simulink model "Simscape_assignment"  (R2022a)
settings: Solver=VariableStepAuto  StartTime=0.0  StopTime=10.0  RelTol=1e-3
values from neighbouring files (symbols this model uses):
  c1 = 1500    [main.m]
  c2 = c1    (= 1500)    [main.m]
  V = 20/3.6    (= 5.55555555556)    [main.m]
libraries: fl_lib x20, nesl_utility x11, sdl_lib x4, cstblocks x1, motdrv_lib x1
settings Model: Creator=s393429  LastModifiedBy=s393429

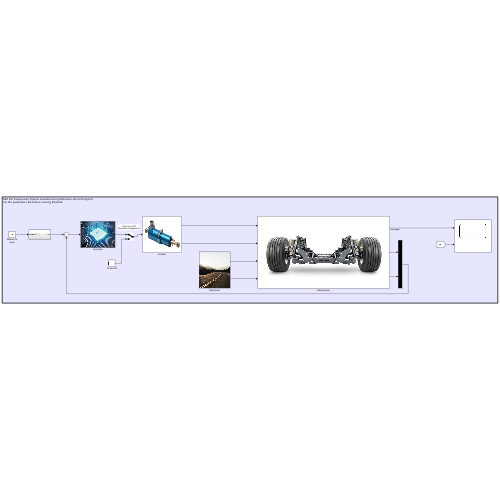
[thumbnail: Simulink's stored preview of the top-level diagram]
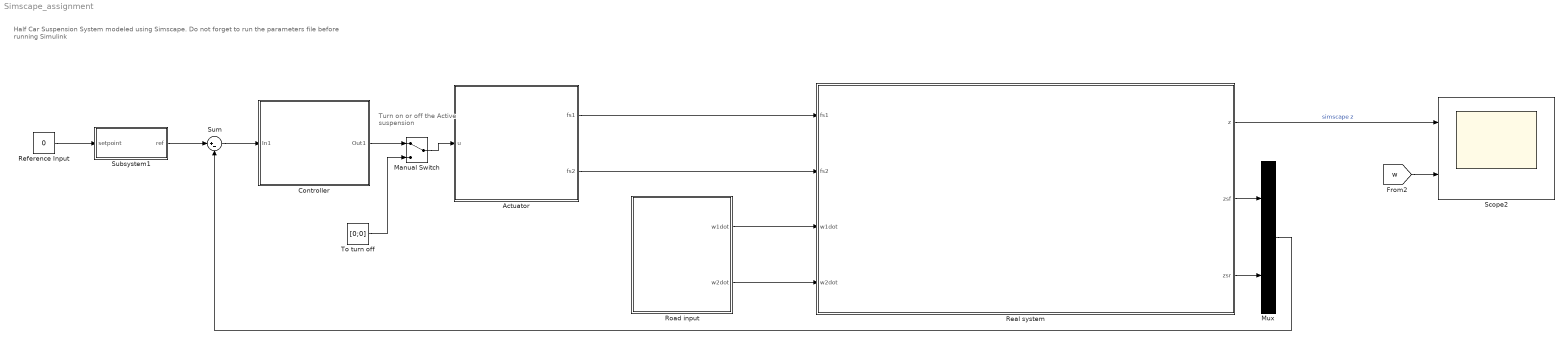
== system Simscape_assignment ==
  note: Half Car Suspension System modeled using Simscape. Do not forget to
      | run the parameters file before running Simulink
  note: Turn on or off
      | the Active suspension
  Actuator : Subsystem
      mask Display: image('actuator.jpg'); % Use "Edit Image" on toolstrip to change.
  Controller : Subsystem
      mask Display: image('cu.jpg'); % Use "Edit Image" on toolstrip to change.
  Manual Switch : ManualSwitch
  Mux : Mux  Inputs=2
  Real system : Subsystem
      mask Display: image('susp.jpg'); % Use "Edit Image" on toolstrip to change.
  Reference Input : Constant  Value=0
  Road input : Subsystem
      mask Display: image('road.jpg'); % Use "Edit Image" on toolstrip to change.
  Scope2 : Scope  NumInputPorts=2
  Subsystem1 : Subsystem
  Sum : Sum  Inputs=|+-
  To turn off : Constant  Value=[0;0]
  wires:
  Actuator/2(fs2) -> Real system/2(fs2)
  Actuator/1(fs1) -> Real system/1(fs1)
  [w] -> Scope2/2
  Real system/2(zsf) -> Mux/1
  Reference Input/1 -> Subsystem1/1(setpoint)
  Real system/3(zsr) -> Mux/2
  Road input/1(w1dot) -> Real system/3(w1dot)
  Sum/1 -> Controller/1(In1)
  Mux/1 -> Sum/2
  Subsystem1/1(ref) -> Sum/1
  Road input/2(w2dot) -> Real system/4(w2dot)
  Real system/1(z) -> Scope2/1  "simscape z"
  Controller/1(Out1) -> Manual Switch/1
  Manual Switch/1 -> Actuator/1(u)
  To turn off/1 -> Manual Switch/2

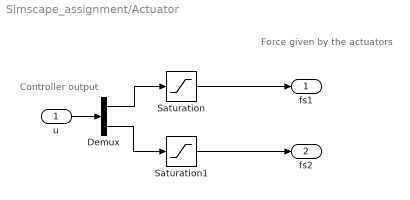
== system Simscape_assignment/Actuator ==
  note: Force given by
      | the actuators
  note: Controller output
  u : Inport
  Demux : Demux  Outputs=2
  Saturation : Saturate  UpperLimit=1e4  LowerLimit=-1e4
  Saturation1 : Saturate  UpperLimit=1e4  LowerLimit=-1e4
  fs1 : Outport
  fs2 : Outport  Port=2
  wires:
  u/1 -> Demux/1
  Demux/1 -> Saturation/1
  Saturation/1 -> fs1/1
  Demux/2 -> Saturation1/1
  Saturation1/1 -> fs2/1

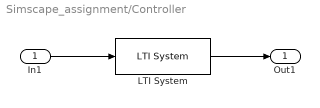
== system Simscape_assignment/Controller ==
  In1 : Inport
  LTI System : cstblocks/LTI System  sys=C  IC=[]
  Out1 : Outport
  wires:
  In1/1 -> LTI System/1
  LTI System/1 -> Out1/1

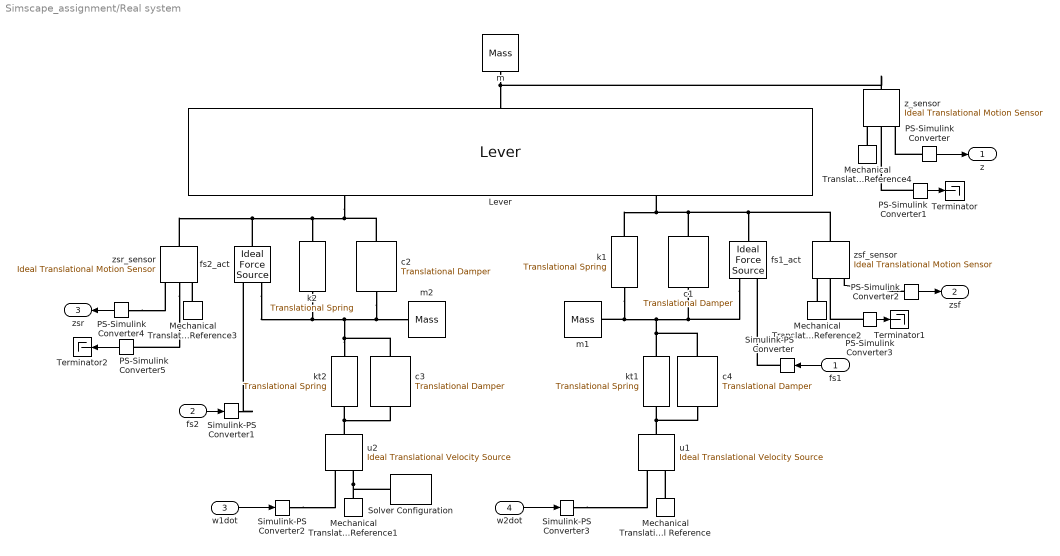
== system Simscape_assignment/Real system ==
  fs1 : Inport
  fs2 : Inport  Port=2
  w1dot : Inport  Port=3
  w2dot : Inport  Port=4
  Lever : fl_lib/Mechanical/Mechanisms/Lever  arm_AC=ar m  arm_BC=af m  f_A_specify=off  f_A_priority=None  f_A=0 N  f_A_nominal_specify=off  f_A_nominal_unit=N  f_A_nominal_value=1  f_B_specify=off  f_B_priority=None  f_B=0 N  f_B_nominal_specify=off  f_B_nominal_unit=N  f_B_nominal_value=1  f_C_specify=off  f_C_priority=None  f_C=0 N  f_C_nominal_specify=off  f_C_nominal_unit=N  f_C_nominal_value=1
      settings: SourceProductBaseCode=PW,SS,VE  InternalSimscapePortConfiguration="{\"Bottom\":[],\"Left\":[{\"id\":\"A\",\"label\":\"A\",\"type\":\"foundation.mechanical.translational.translational\"},{\"id\":\"B\",\"label\":\"B\",\"type\":\"foundation.mechanical.translational.translational\"}],\"Right\":[{\"id\":\"C\",\"label\":\"C\",\"type\":\"foundation.mechanical.translational.translational\"}],\"Top\":[]}"
  Mechanical Translational Reference{,1..4} (5 alike) : fl_lib/Mechanical/Translational Elements/Mechanical Translational Reference
      settings: SourceProductBaseCode=PW,SS,VE
  PS-Simulink Converter : nesl_utility/PS-Simulink Converter  PhysicalDomain=network_engine_domain  SubClassName=ps_output  LeftPortType=input  RightPortType=output  PseudoPeriodic=off  Frequencies=[]  VectorFormat=inherit  Unit=m  AffineConversion=off
      settings: SourceProductBaseCode=SS,PW,VE
  PS-Simulink Converter1 : nesl_utility/PS-Simulink Converter  PhysicalDomain=network_engine_domain  SubClassName=ps_output  LeftPortType=input  RightPortType=output  PseudoPeriodic=off  Frequencies=[]  VectorFormat=inherit  Unit=m/s  AffineConversion=off
      settings: SourceProductBaseCode=SS,PW,VE
  PS-Simulink Converter2 : nesl_utility/PS-Simulink Converter  PhysicalDomain=network_engine_domain  SubClassName=ps_output  LeftPortType=input  RightPortType=output  PseudoPeriodic=off  Frequencies=[]  VectorFormat=inherit  Unit=m  AffineConversion=off
      settings: SourceProductBaseCode=SS,PW,VE
  PS-Simulink Converter3 : nesl_utility/PS-Simulink Converter  PhysicalDomain=network_engine_domain  SubClassName=ps_output  LeftPortType=input  RightPortType=output  PseudoPeriodic=off  Frequencies=[]  VectorFormat=inherit  Unit=m/s  AffineConversion=off
      settings: SourceProductBaseCode=SS,PW,VE
  PS-Simulink Converter4 : nesl_utility/PS-Simulink Converter  PhysicalDomain=network_engine_domain  SubClassName=ps_output  LeftPortType=input  RightPortType=output  PseudoPeriodic=off  Frequencies=[]  VectorFormat=inherit  Unit=m  AffineConversion=off
      settings: SourceProductBaseCode=SS,PW,VE
  PS-Simulink Converter5 : nesl_utility/PS-Simulink Converter  PhysicalDomain=network_engine_domain  SubClassName=ps_output  LeftPortType=input  RightPortType=output  PseudoPeriodic=off  Frequencies=[]  VectorFormat=inherit  Unit=m/s  AffineConversion=off
      settings: SourceProductBaseCode=SS,PW,VE
  Simulink-PS Converter : nesl_utility/Simulink-PS Converter  PhysicalDomain=network_engine_domain  SubClassName=ps_input  LeftPortType=input  RightPortType=output  PseudoPeriodic=off  Frequencies=[]  NoiseDistribution=none  NoiseParameters=[]  Unit=N  AffineConversion=off  FilteringAndDerivatives=provide  SimscapeFilterOrder=1  InputFilterTimeConstant=0.001  UdotUserProvided=0
      settings: SourceProductBaseCode=SS,PW,VE
  Simulink-PS Converter1 : nesl_utility/Simulink-PS Converter  PhysicalDomain=network_engine_domain  SubClassName=ps_input  LeftPortType=input  RightPortType=output  PseudoPeriodic=off  Frequencies=[]  NoiseDistribution=none  NoiseParameters=[]  Unit=N  AffineConversion=off  FilteringAndDerivatives=provide  SimscapeFilterOrder=1  InputFilterTimeConstant=0.001  UdotUserProvided=0
      settings: SourceProductBaseCode=SS,PW,VE
  Simulink-PS Converter2 : nesl_utility/Simulink-PS Converter  PhysicalDomain=network_engine_domain  SubClassName=ps_input  LeftPortType=input  RightPortType=output  PseudoPeriodic=off  Frequencies=[]  NoiseDistribution=none  NoiseParameters=[]  Unit=m/s  AffineConversion=off  FilteringAndDerivatives=provide  SimscapeFilterOrder=1  InputFilterTimeConstant=0.001  UdotUserProvided=0
      settings: SourceProductBaseCode=SS,PW,VE
  Simulink-PS Converter3 : nesl_utility/Simulink-PS Converter  PhysicalDomain=network_engine_domain  SubClassName=ps_input  LeftPortType=input  RightPortType=output  PseudoPeriodic=off  Frequencies=[]  NoiseDistribution=none  NoiseParameters=[]  Unit=m/s  AffineConversion=off  FilteringAndDerivatives=provide  SimscapeFilterOrder=1  InputFilterTimeConstant=0.001  UdotUserProvided=0
      settings: SourceProductBaseCode=SS,PW,VE
  Solver Configuration : nesl_utility/Solver Configuration  PhysicalDomain=network_engine_domain  SubClassName=solver  LeftPortType=input  RightPortType=generic  Tones=[]  Harmonics=[]  SimulateNoise=off  Profile=off  UseLocalSampling=off  EnableSwitchedLinearOptims=on  FrequencyDomain=off  UseCCode=off  RelTol=0.001  AbsTol=0.001  MinStep=1e-09  ToWorkspace=off  RevertToSquareIcSolve=off  NumHomotopyIterations=100  PhasorMode=off  PhasorModeNumHarmonics=1  IndexReductionMethod=DerivativeReplacement  DoDC=off  ResidualTolerance=1e-09  UseLocalSolver=off  LocalSolverChoice=NE_BACKWARD_EULER_ADVANCER  LocalSolverSampleTime=0.001  DoFixedCost=off  MaxNonlinIter=3  MaxModeIter=2  ComputeImpulses=off  ImpulseIterations=2  LinearAlgebra=auto  LinearAlgebraNumThread=0  EquationFormulation=NE_TIME_EF  DelaysMemoryBudget=1024  AutomaticFiltering=on  FilteringTimeConstant=0.001  PartitionStorageMethod=AS_NEEDED  PartitionMemoryBudget=1024  PartitionMethod=ROBUST
      settings: SourceProductBaseCode=SS,PW,VE
  Terminator : Terminator
  Terminator1 : Terminator
  Terminator2 : Terminator
  c1 : sdl_lib/Couplings & Drives/Springs & Dampers/Translational Damper  D=c1 N*s/m  enable_faults=simscape.enum.onoff.off  b_fault=1e6 N*s/m  temporal_fault=simscape.enum.onoff.off  fault_time=5 s  shock_fault=simscape.enum.onoff.off  acceleration_limit=100 m/s^2  shock_limit=1  report_fault=simscape.enum.assert.action.none  thermal_port=simscape.enum.thermaleffects.omit  thermal_mass=50 kJ/K  temperature_specify=off  temperature_priority=High  temperature=300 K  temperature_nominal_specify=off  temperature_nominal_unit=K  temperature_nominal_value=1
      settings: SourceProductBaseCode=LD
  c2 : sdl_lib/Couplings & Drives/Springs & Dampers/Translational Damper  D=c2 N*s/m  enable_faults=simscape.enum.onoff.off  b_fault=1e6 N*s/m  temporal_fault=simscape.enum.onoff.off  fault_time=5 s  shock_fault=simscape.enum.onoff.off  acceleration_limit=100 m/s^2  shock_limit=1  report_fault=simscape.enum.assert.action.none  thermal_port=simscape.enum.thermaleffects.omit  thermal_mass=50 kJ/K  temperature_specify=off  temperature_priority=High  temperature=300 K  temperature_nominal_specify=off  temperature_nominal_unit=K  temperature_nominal_value=1
      settings: SourceProductBaseCode=LD
  c3 : sdl_lib/Couplings & Drives/Springs & Dampers/Translational Damper  D=1000 N*s/m  enable_faults=simscape.enum.onoff.off  b_fault=1e6 N*s/m  temporal_fault=simscape.enum.onoff.off  fault_time=5 s  shock_fault=simscape.enum.onoff.off  acceleration_limit=100 m/s^2  shock_limit=1  report_fault=simscape.enum.assert.action.none  thermal_port=simscape.enum.thermaleffects.omit  thermal_mass=50 kJ/K  temperature_specify=off  temperature_priority=High  temperature=300 K  temperature_nominal_specify=off  temperature_nominal_unit=K  temperature_nominal_value=1
      settings: SourceProductBaseCode=LD
  c4 : sdl_lib/Couplings & Drives/Springs & Dampers/Translational Damper  D=1000 N*s/m  enable_faults=simscape.enum.onoff.off  b_fault=1e6 N*s/m  temporal_fault=simscape.enum.onoff.off  fault_time=5 s  shock_fault=simscape.enum.onoff.off  acceleration_limit=100 m/s^2  shock_limit=1  report_fault=simscape.enum.assert.action.none  thermal_port=simscape.enum.thermaleffects.omit  thermal_mass=50 kJ/K  temperature_specify=off  temperature_priority=High  temperature=300 K  temperature_nominal_specify=off  temperature_nominal_unit=K  temperature_nominal_value=1
      settings: SourceProductBaseCode=LD
  fs1_act : fl_lib/Mechanical/Mechanical Sources/Ideal Force Source
      settings: SourceProductBaseCode=PW,SS,VE
  fs2_act : fl_lib/Mechanical/Mechanical Sources/Ideal Force Source
      settings: SourceProductBaseCode=PW,SS,VE
  k1 : fl_lib/Mechanical/Translational Elements/Translational Spring  spr_rate=k1 N/m  v_specify=off  v_priority=None  v=0 m/s  v_nominal_specify=off  v_nominal_unit=m/s  v_nominal_value=1  f_specify=off  f_priority=None  f=0 N  f_nominal_specify=off  f_nominal_unit=N  f_nominal_value=1  x_specify=off  x_priority=High  x=0 m  x_nominal_specify=off  x_nominal_unit=m  x_nominal_value=1
      settings: SourceProductBaseCode=PW,SS,VE
  k2 : fl_lib/Mechanical/Translational Elements/Translational Spring  spr_rate=k2 N/m  v_specify=off  v_priority=None  v=0 m/s  v_nominal_specify=off  v_nominal_unit=m/s  v_nominal_value=1  f_specify=off  f_priority=None  f=0 N  f_nominal_specify=off  f_nominal_unit=N  f_nominal_value=1  x_specify=off  x_priority=High  x=0 m  x_nominal_specify=off  x_nominal_unit=m  x_nominal_value=1
      settings: SourceProductBaseCode=PW,SS,VE
  kt1 : fl_lib/Mechanical/Translational Elements/Translational Spring  spr_rate=kt1 N/m  v_specify=off  v_priority=None  v=0 m/s  v_nominal_specify=off  v_nominal_unit=m/s  v_nominal_value=1  f_specify=off  f_priority=None  f=0 N  f_nominal_specify=off  f_nominal_unit=N  f_nominal_value=1  x_specify=off  x_priority=High  x=0 m  x_nominal_specify=off  x_nominal_unit=m  x_nominal_value=1
      settings: SourceProductBaseCode=PW,SS,VE
  kt2 : fl_lib/Mechanical/Translational Elements/Translational Spring  spr_rate=kt2 N/m  v_specify=off  v_priority=None  v=0 m/s  v_nominal_specify=off  v_nominal_unit=m/s  v_nominal_value=1  f_specify=off  f_priority=None  f=0 N  f_nominal_specify=off  f_nominal_unit=N  f_nominal_value=1  x_specify=off  x_priority=High  x=0 m  x_nominal_specify=off  x_nominal_unit=m  x_nominal_value=1
      settings: SourceProductBaseCode=PW,SS,VE
  m : fl_lib/Mechanical/Translational Elements/Mass  mass=m kg  num_ports=foundation.enum.numPorts2.one  v_specify=off  v_priority=High  v=0 m/s  v_nominal_specify=off  v_nominal_unit=m/s  v_nominal_value=1  f_specify=off  f_priority=None  f=0 N  f_nominal_specify=off  f_nominal_unit=N  f_nominal_value=1
      settings: SourceProductBaseCode=PW,SS,VE
  m1 : fl_lib/Mechanical/Translational Elements/Mass  mass=m1 kg  num_ports=foundation.enum.numPorts2.one  v_specify=off  v_priority=High  v=0 m/s  v_nominal_specify=off  v_nominal_unit=m/s  v_nominal_value=1  f_specify=off  f_priority=None  f=0 N  f_nominal_specify=off  f_nominal_unit=N  f_nominal_value=1
      settings: SourceProductBaseCode=PW,SS,VE
  m2 : fl_lib/Mechanical/Translational Elements/Mass  mass=m2 kg  num_ports=foundation.enum.numPorts2.one  v_specify=off  v_priority=High  v=0 m/s  v_nominal_specify=off  v_nominal_unit=m/s  v_nominal_value=1  f_specify=off  f_priority=None  f=0 N  f_nominal_specify=off  f_nominal_unit=N  f_nominal_value=1
      settings: SourceProductBaseCode=PW,SS,VE
  u1 : fl_lib/Mechanical/Mechanical Sources/Ideal Translational Velocity Source
      settings: SourceProductBaseCode=PW,SS,VE
  u2 : fl_lib/Mechanical/Mechanical Sources/Ideal Translational Velocity Source
      settings: SourceProductBaseCode=PW,SS,VE
  z_sensor : fl_lib/Mechanical/Mechanical Sensors/Ideal Translational Motion Sensor  offset=0 m
      settings: SourceProductBaseCode=PW,SS,VE
  zsf_sensor : fl_lib/Mechanical/Mechanical Sensors/Ideal Translational Motion Sensor  offset=0 m
      settings: SourceProductBaseCode=PW,SS,VE
  zsr_sensor : fl_lib/Mechanical/Mechanical Sensors/Ideal Translational Motion Sensor  offset=0 m
      settings: SourceProductBaseCode=PW,SS,VE
  z : Outport
  zsf : Outport  Port=2
  zsr : Outport  Port=3
  wires:
  PS-Simulink Converter1/1 -> Terminator/1
  PS-Simulink Converter/1 -> z/1
  PS-Simulink Converter2/1 -> zsf/1
  PS-Simulink Converter3/1 -> Terminator1/1
  PS-Simulink Converter4/1 -> zsr/1
  PS-Simulink Converter5/1 -> Terminator2/1
  fs1/1 -> Simulink-PS Converter/1
  fs2/1 -> Simulink-PS Converter1/1
  w1dot/1 -> Simulink-PS Converter2/1
  w2dot/1 -> Simulink-PS Converter3/1
  connections:
  Lever/LConn1 -- fs2_act/LConn1 -- zsr_sensor/LConn1 -- k2/LConn1 -- c2/LConn1
  Simulink-PS Converter1/RConn1 -- fs2_act/RConn1
  k1/RConn1 -- m1/LConn1 -- fs1_act/RConn2 -- c1/RConn1 -- kt1/LConn1 -- c4/LConn1
  PS-Simulink Converter2/LConn1 -- zsf_sensor/RConn3
  PS-Simulink Converter/LConn1 -- z_sensor/RConn3
  k1/LConn1 -- zsf_sensor/LConn1 -- fs1_act/LConn1 -- c1/LConn1 -- Lever/LConn2
  kt2/LConn1 -- k2/RConn1 -- fs2_act/RConn2 -- m2/LConn1 -- c2/RConn1 -- c3/LConn1
  Mechanical Translational Reference1/LConn1 -- Solver Configuration/RConn1 -- u2/RConn2
  Simulink-PS Converter/RConn1 -- fs1_act/RConn1
  m/LConn1 -- z_sensor/LConn1 -- Lever/RConn1
  Mechanical Translational Reference2/LConn1 -- zsf_sensor/RConn1
  kt1/RConn1 -- u1/LConn1 -- c4/RConn1
  Mechanical Translational Reference4/LConn1 -- z_sensor/RConn1
  kt2/RConn1 -- u2/LConn1 -- c3/RConn1
  Mechanical Translational Reference/LConn1 -- u1/RConn2
  PS-Simulink Converter1/LConn1 -- z_sensor/RConn2
  Mechanical Translational Reference3/LConn1 -- zsr_sensor/RConn1
  PS-Simulink Converter3/LConn1 -- zsf_sensor/RConn2
  PS-Simulink Converter4/LConn1 -- zsr_sensor/RConn3
  zsr_sensor/RConn2 -- PS-Simulink Converter5/LConn1
  Simulink-PS Converter2/RConn1 -- u2/RConn1
  Simulink-PS Converter3/RConn1 -- u1/RConn1

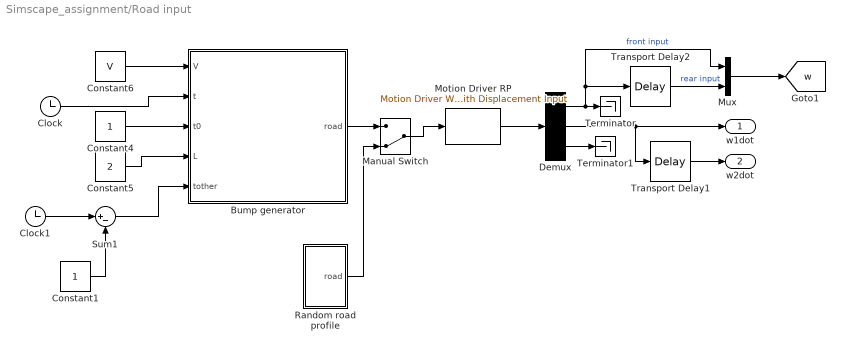
== system Simscape_assignment/Road input ==
  Bump generator : MATLAB Function  TreatAsAtomicUnit=on
  Clock : Clock
  Clock1 : Clock
  Constant1 : Constant
  Constant4 : Constant
  Constant5 : Constant  Value=2
  Constant6 : Constant  Value=V
  Demux : Demux  Outputs=3
  Manual Switch : ManualSwitch  CurrentSetting=0
  Motion Driver RP : motdrv_lib/Motion Driver With Displacement Input  InitialDisplacement=0  InitialVelocity=0  TimeConstant=1/128
  Mux : Mux  Inputs=2
  Random road profile : Subsystem
  Sum1 : Sum  Inputs=|+-
  Terminator : Terminator
  Terminator1 : Terminator
  Transport Delay1 : TransportDelay  DelayTime=0.1625
  Transport Delay2 : TransportDelay  DelayTime=0.1625
  w1dot : Outport
  w2dot : Outport  Port=2
  tag scope: w=global
  wires:
  Constant4/1 -> Bump generator/3(t0)
  Sum1/1 -> Bump generator/5(tother)
  Constant1/1 -> Sum1/2
  Constant5/1 -> Bump generator/4(L)
  Clock/1 -> Bump generator/2(t)
  Clock1/1 -> Sum1/1
  Constant6/1 -> Bump generator/1(V)
  Motion Driver RP/1 -> Demux/1
  Demux/2 -> Transport Delay1/1, w1dot/1
  Transport Delay1/1 -> w2dot/1
  Demux/3 -> Terminator1/1
  Bump generator/1(road) -> Manual Switch/1
  Manual Switch/1 -> Motion Driver RP/1
  Random road profile/1(road) -> Manual Switch/2
  Demux/1 -> Transport Delay2/1, Mux/1, Terminator/1  "front input"
  Transport Delay2/1 -> Mux/2  "rear input"
  Mux/1 -> [w]

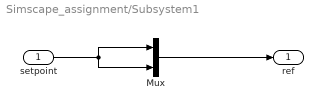
== system Simscape_assignment/Subsystem1 ==
  setpoint : Inport
  Mux : Mux  Inputs=2
  ref : Outport
  wires:
  setpoint/1 -> Mux/1, Mux/2
  Mux/1 -> ref/1

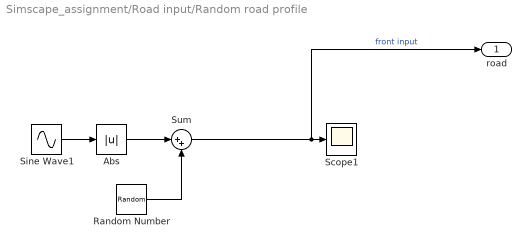
== system Simscape_assignment/Road input/Random road profile ==
  Abs : Abs  SaturateOnIntegerOverflow=off
  Random Number : RandomNumber  Variance=.0001  SampleTime=0.01
  Scope1 : Scope
  Sine Wave1 : Sin  Amplitude=.05  Frequency=5  SampleTime=0
  Sum : Sum  Inputs=|++
  road : Outport
  wires:
  Sine Wave1/1 -> Abs/1
  Abs/1 -> Sum/1
  Sum/1 -> road/1, Scope1/1  "front input"
  Random Number/1 -> Sum/2

== matlab function Simscape_assignment/Road input/Bump generator ==
  data: V input; road output; t input; t0 input; L input; tother input
function road = fcn(V, t, t0, L, tother)


if t>t0 && t<=t0+L/V
        road = -1/2*0.30*(cos(2*pi*V*tother/L)-1);
else 
    road = 0;
end

end
